simulink model "Full_sim"  (Simulink 7.8)
settings: Solver=FixedStepDiscrete  StartTime=0.0  StopTime=1000  FixedStep=.01  RelTol=1e-3
InitFcn:
  | missions
  | common
  | physical_constants
  | simulation_constants
  | l2plus
libraries: simulink x1
settings Model: Creator=Administrator  LastModifiedBy=Bryant  ExtModeAutoUpdateStatusClock=off  BufferReuse=off
settings DataIOCC: LimitDataPoints=off  MaxDataPoints=1  SaveOutput=off  SignalLogging=off
settings OptimizationCC: BlockReduction=off  InlineParams=on  InlineInvariantSignals=on  BufferReuse=off  InitFltsAndDblsToZero=on  EfficientMapNaN2IntZero=off  LifeSpan=30  SimCompilerOptimization=On
settings DebuggingCC: ReadBeforeWriteMsg=DisableAll  SaveWithParameterizedLinksMsg=none  UnderspecifiedInitializationDetection=Simplified  UniqueDataStoreMsg=error  AssertControl=DisableAll
settings HardwareCC: ProdHWDeviceType=Generic->Unspecified (assume 32-bit Generic)  TargetIntDivRoundTo=Zero  TargetEndianess=LittleEndian  TargetHWDeviceType=Microchip->dsPIC
settings SFSimCC: SimParseCustomCode=off
settings CodeAppCC: MaxIdLength=128

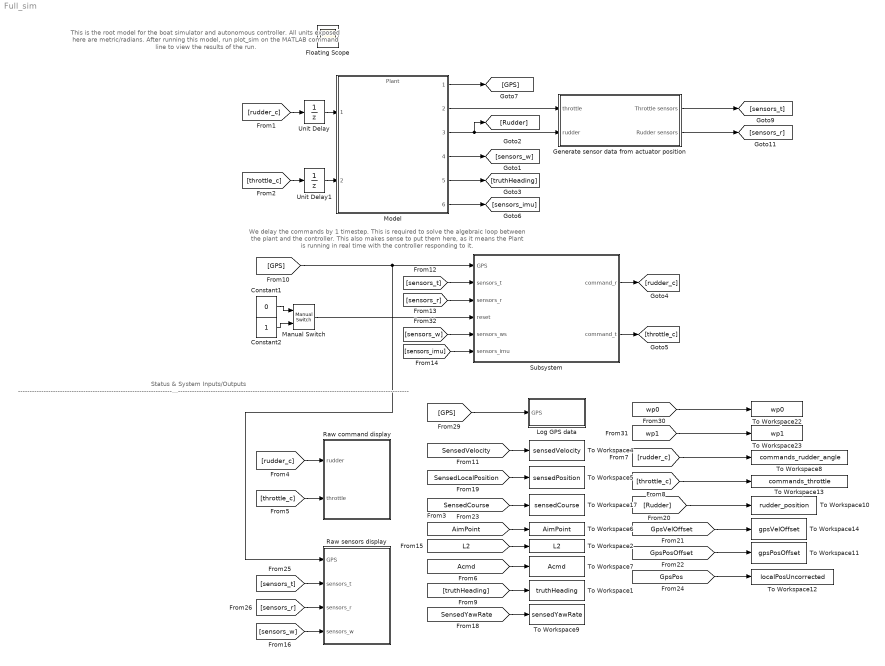
== system Full_sim ==
  note: This is the root model for the boat simulator and autonomous controller. All
      | units exposed here are metric/radians.
      |
      | After running this model, run plot_sim on the MATLAB command line to
      | view the results of the run.
  note: Status & System Inputs/Outputs
      | ---------------------------------------------------------------------------------------------------------------------------------------------------------------------------------------------------------------------------------------------------------
  note: We delay the commands by 1 timestep. This is required to solve the algebraic loop between the plant and the controller.
      | This also makes sense to put them here, as it means the Plant is running in real time with the controller responding to it.
  Constant1 : Constant  Value=0  OutDataTypeStr=boolean  SampleTime=Inf
  Constant2 : Constant  OutDataTypeStr=boolean  SampleTime=Inf
  Generate sensor data from actuator position : Subsystem
  Log GPS data : Subsystem
  Manual Switch : simulink/Signal Routing/Manual Switch  sw=1  action=0  varsize=off
  Model : ModelReference  ModelNameDialog=Plant  SimulationMode=Normal  ModelReferenceVersion=1.64  CopyOfModelName=Plant  DefaultDataLogging=on
  Raw command display : Subsystem
  Raw sensors display : Subsystem
  Subsystem : Subsystem
  To Workspace1 : ToWorkspace  VariableName=truthHeading  SampleTime=-1  SaveFormat=Array
  To Workspace10 : ToWorkspace  VariableName=rudder_position  SampleTime=-1  SaveFormat=Array
  To Workspace11 : ToWorkspace  VariableName=gpsPosOffset  SampleTime=-1  SaveFormat=Array
  To Workspace12 : ToWorkspace  VariableName=localPosUncorrected  SampleTime=-1  SaveFormat=Array
  To Workspace13 : ToWorkspace  VariableName=commands_throttle  SampleTime=-1  SaveFormat=Array
  To Workspace14 : ToWorkspace  VariableName=gpsVelOffset  SampleTime=-1  SaveFormat=Array
  To Workspace17 : ToWorkspace  VariableName=sensedCourse  SampleTime=-1  SaveFormat=Array
  To Workspace2 : ToWorkspace  VariableName=L2  SampleTime=-1  SaveFormat=Array
  To Workspace22 : ToWorkspace  VariableName=wp0  SampleTime=-1  SaveFormat=Array
  To Workspace23 : ToWorkspace  VariableName=wp1  SampleTime=-1  SaveFormat=Array
  To Workspace4 : ToWorkspace  VariableName=sensedVelocity  SampleTime=-1  SaveFormat=Array
  To Workspace5 : ToWorkspace  VariableName=sensedPosition  SampleTime=-1  SaveFormat=Array
  To Workspace6 : ToWorkspace  VariableName=AimPoint  SampleTime=-1  SaveFormat=Array
  To Workspace7 : ToWorkspace  VariableName=Acmd  SampleTime=-1  SaveFormat=Array
  To Workspace8 : ToWorkspace  VariableName=commands_rudder_angle  SampleTime=-1  SaveFormat=Array
  To Workspace9 : ToWorkspace  VariableName=sensedYawRate  SampleTime=-1  SaveFormat=Array
  Unit Delay : UnitDelay  SampleTime=-1
  Unit Delay1 : UnitDelay  SampleTime=-1
  Floating Scope : Scope
      settings: Floating=on
  wires:
  Model/3 -> Generate sensor data from actuator position/2(rudder), [Rudder]
  Subsystem/1(command_r) -> [rudder_c]
  Subsystem/2(command_t) -> [throttle_c]
  [rudder_c] -> Unit Delay/1
  Model/1 -> [GPS]
  Model/2 -> Generate sensor data from actuator position/1(throttle)
  [sensors_r] -> Subsystem/3(sensors_r)
  [sensors_t] -> Subsystem/2(sensors_t)
  Constant1/1 -> Manual Switch/1
  Constant2/1 -> Manual Switch/2
  Manual Switch/1 -> Subsystem/4(reset)
  [GPS] -> Subsystem/1(GPS), Raw sensors display/1(GPS)
  Model/4 -> [sensors_w]
  [sensors_w] -> Subsystem/5(sensors_ws)
  [rudder_c] -> Raw command display/1(rudder)
  [throttle_c] -> Raw command display/2(throttle)
  [sensors_t] -> Raw sensors display/2(sensors_t)
  [sensors_r] -> Raw sensors display/3(sensors_r)
  [Rudder] -> To Workspace10/1
  [throttle_c] -> To Workspace13/1
  [rudder_c] -> To Workspace8/1
  [SensedVelocity] -> To Workspace4/1
  [SensedLocalPosition] -> To Workspace5/1
  [SensedCourse] -> To Workspace17/1
  [GPS] -> Log GPS data/1(GPS)
  [wp0] -> To Workspace22/1
  [wp1] -> To Workspace23/1
  Unit Delay/1 -> Model/1
  Unit Delay1/1 -> Model/2
  [AimPoint] -> To Workspace6/1
  [Acmd] -> To Workspace7/1
  Generate sensor data from actuator position/1(Throttle sensors) -> [sensors_t]
  Generate sensor data from actuator position/2(Rudder sensors) -> [sensors_r]
  Model/5 -> [truthHeading]
  [truthHeading] -> To Workspace1/1
  Model/6 -> [sensors_imu]
  [sensors_imu] -> Subsystem/6(sensors_imu)
  [L2] -> To Workspace2/1
  [sensors_w] -> Raw sensors display/4(sensors_w)
  [SensedYawRate] -> To Workspace9/1
  [GpsVelOffset] -> To Workspace14/1
  [GpsPosOffset] -> To Workspace11/1
  [GpsPos] -> To Workspace12/1
  [throttle_c] -> Unit Delay1/1

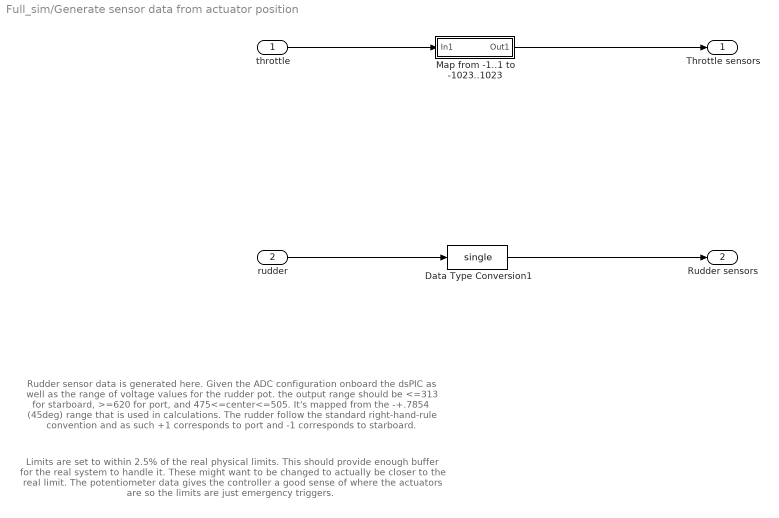
== system Full_sim/Generate sensor data from actuator position ==
  note: Rudder sensor data is generated here. Given the ADC configuration onboard the dsPIC
      | as well as the range of voltage values for the rudder pot. the output range should be
      | <=313 for starboard, >=620 for port, and 475<=center<=505. It's mapped from the -+.7854
      | (45deg) range that is used in calculations. The rudder follow the standard right-hand-rule
      | convention and as such +1 corresponds to port and -1 corresponds to starboard.
  note: Limits are set to within 2.5% of the real physical limits. This should
      | provide enough buffer for the real system to handle it. These might want to be changed
      | to actually be closer to the real limit. The potentiometer data gives the controller a good
      | sense of where the actuators are so the limits are just emergency triggers.
  throttle : Inport
  rudder : Inport  Port=2
  Data Type Conversion1 : DataTypeConversion  OutDataTypeStr=single  RndMeth=Simplest
  Map from -1..1 to -1023..1023 : Subsystem
  Throttle sensors : Outport
  Rudder sensors : Outport  Port=2
  wires:
  throttle/1 -> Map from -1..1 to -1023..1023/1(In1)
  rudder/1 -> Data Type Conversion1/1
  Map from -1..1 to -1023..1023/1(Out1) -> Throttle sensors/1
  Data Type Conversion1/1 -> Rudder sensors/1

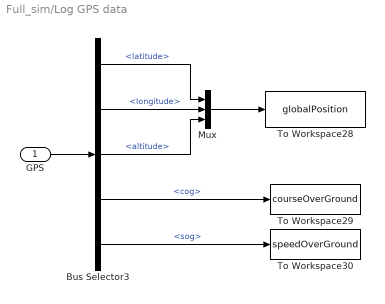
== system Full_sim/Log GPS data ==
  GPS : Inport
  Bus Selector3 : BusSelector  OutputSignals=latitude,longitude,altitude,cog,sog
  Mux : Mux  Inputs=3
  To Workspace28 : ToWorkspace  VariableName=globalPosition  SampleTime=-1  SaveFormat=Array
  To Workspace29 : ToWorkspace  VariableName=courseOverGround  SampleTime=-1  SaveFormat=Array
  To Workspace30 : ToWorkspace  VariableName=speedOverGround  SampleTime=-1  SaveFormat=Array
  wires:
  Mux/1 -> To Workspace28/1
  Bus Selector3/1 -> Mux/1  "<latitude>"
  Bus Selector3/2 -> Mux/2  "<longitude>"
  Bus Selector3/3 -> Mux/3  "<altitude>"
  Bus Selector3/4 -> To Workspace29/1  "<cog>"
  Bus Selector3/5 -> To Workspace30/1  "<sog>"
  GPS/1 -> Bus Selector3/1

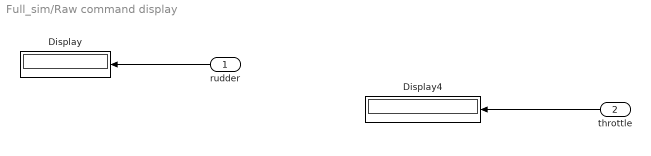
== system Full_sim/Raw command display ==
  rudder : Inport
  throttle : Inport  Port=2
  Display : Display
  Display4 : Display
      settings: Format=hex (Stored Integer)
  wires:
  throttle/1 -> Display4/1
  rudder/1 -> Display/1

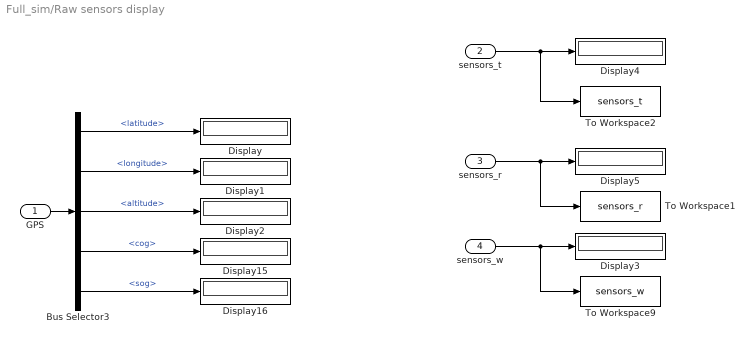
== system Full_sim/Raw sensors display ==
  GPS : Inport
  sensors_t : Inport  Port=2
  sensors_r : Inport  Port=3
  sensors_w : Inport  Port=4
  Bus Selector3 : BusSelector  OutputSignals=latitude,longitude,altitude,cog,sog
  Display{,1..5,15..16} (8 alike) : Display
  To Workspace1 : ToWorkspace  VariableName=sensors_r  SampleTime=-1  SaveFormat=Array
  To Workspace2 : ToWorkspace  VariableName=sensors_t  SampleTime=-1  SaveFormat=Array
  To Workspace9 : ToWorkspace  VariableName=sensors_w  SampleTime=-1  SaveFormat=Array
  wires:
  Bus Selector3/1 -> Display/1  "<latitude>"
  Bus Selector3/2 -> Display1/1  "<longitude>"
  Bus Selector3/3 -> Display2/1  "<altitude>"
  GPS/1 -> Bus Selector3/1
  sensors_t/1 -> Display4/1, To Workspace2/1
  sensors_r/1 -> Display5/1, To Workspace1/1
  Bus Selector3/4 -> Display15/1  "<cog>"
  Bus Selector3/5 -> Display16/1  "<sog>"
  sensors_w/1 -> Display3/1, To Workspace9/1

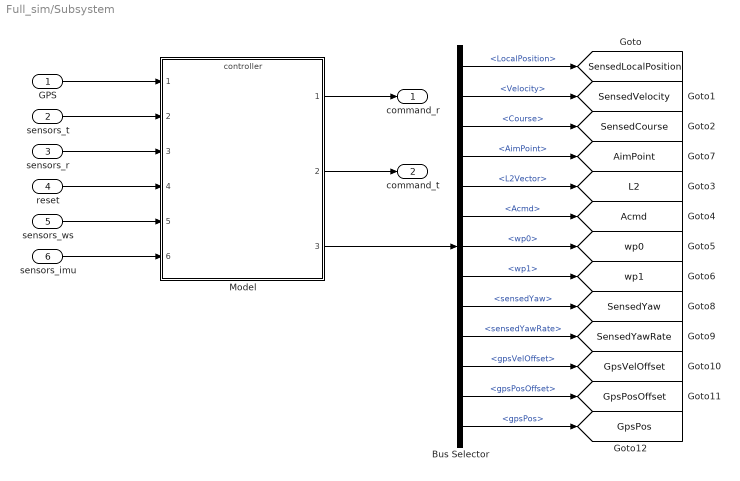
== system Full_sim/Subsystem ==
  GPS : Inport
  sensors_t : Inport  Port=2
  sensors_r : Inport  Port=3
  reset : Inport  Port=4
  sensors_ws : Inport  Port=5
  sensors_imu : Inport  Port=6
  Bus Selector : BusSelector  OutputSignals=LocalPosition,Velocity,Course,AimPoint,L2Vector,Acmd,wp0,wp1,sensedYaw,sensedYawRate,gpsVelOffset,gpsPosOffset,gpsPos
  Model : ModelReference  ModelNameDialog=controller  SimulationMode=Normal  ModelReferenceVersion=1.2834  CopyOfModelName=controller  DefaultDataLogging=on
  command_r : Outport
  command_t : Outport  Port=2
  tag scope: Acmd=global, AimPoint=global, GpsPos=global, GpsPosOffset=global, GpsVelOffset=global, L2=global, SensedCourse=global, SensedLocalPosition=global, SensedVelocity=global, SensedYaw=global, SensedYawRate=global, wp0=global, wp1=global
  wires:
  GPS/1 -> Model/1
  Model/1 -> command_r/1
  sensors_t/1 -> Model/2
  sensors_r/1 -> Model/3
  Model/2 -> command_t/1
  reset/1 -> Model/4
  Model/3 -> Bus Selector/1
  Bus Selector/1 -> [SensedLocalPosition]  "<LocalPosition>"
  Bus Selector/2 -> [SensedVelocity]  "<Velocity>"
  Bus Selector/3 -> [SensedCourse]  "<Course>"
  Bus Selector/5 -> [L2]  "<L2Vector>"
  Bus Selector/6 -> [Acmd]  "<Acmd>"
  Bus Selector/7 -> [wp0]  "<wp0>"
  Bus Selector/8 -> [wp1]  "<wp1>"
  sensors_ws/1 -> Model/5
  sensors_imu/1 -> Model/6
  Bus Selector/4 -> [AimPoint]  "<AimPoint>"
  Bus Selector/9 -> [SensedYaw]  "<sensedYaw>"
  Bus Selector/10 -> [SensedYawRate]  "<sensedYawRate>"
  Bus Selector/11 -> [GpsVelOffset]  "<gpsVelOffset>"
  Bus Selector/12 -> [GpsPosOffset]  "<gpsPosOffset>"
  Bus Selector/13 -> [GpsPos]  "<gpsPos>"

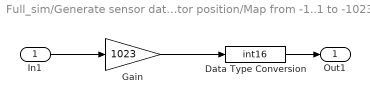
== system Full_sim/Generate sensor data from actuator position/Map from -1..1 to -1023..1023 ==
  In1 : Inport
  Data Type Conversion : DataTypeConversion  OutDataTypeStr=int16  RndMeth=Simplest
  Gain : Gain  Gain=1023
  Out1 : Outport
  wires:
  Gain/1 -> Data Type Conversion/1
  In1/1 -> Gain/1
  Data Type Conversion/1 -> Out1/1
